simulink model "test_8m_0508"  (R2024a)
settings: Solver=FixedStepAuto  StartTime=0.0  StopTime=30  FixedStep=dt  RelTol=1e-3
values from neighbouring files (symbols this model uses):
  attitude_0 = [0; -90;  -0]    [ini_param_8m_0522.m]
  b = 4.0    (= 4)    [ini_param_8m_0522.m]
  cbar = 0.75    [ini_param_8m_0522.m]
  dt = 0.004    [ini_param_8m_0522.m]
  H = 1000    [ini_param_8m_0522.m]
  N_data = [0,200, 491, 804, 1077, 1344, 1559, 1832, 2078, 2318, 2579,            2864, 3117, 3371, 3608.2, 3872, 4055.7, 4291, 4507, 4739, 4935]'    [cal_motor.m]
  N_pwm = 0.01*[0, 5 ,10 ,15 ,20 ,25 ,30 ,35,40, 45 ,50 ,              55 ,60 ,65 ,70, 75, 80 , 85 ,90 ,95 ,100]'    [cal_motor.m]
  pitch_rate_K = 1    [ini_param_8m_0522.m]
  roll_rate_K = 1    [ini_param_8m_0522.m]
  S = 6.0    (= 6)    [ini_param_8m_0522.m]
  Ts = 0.05    [ini_param_8m_0522.m]
  Ts_sur = 0.25    [ini_param_8m_0522.m]
  yaw_rate_K = 1    [ini_param_8m_0522.m]
undefined symbols (not defined in the file or in its folder): sigbuilder_block, UAV
libraries: slpidlib x9, simulink_extras x6, sharedtransform x2, shared6dof x1
(part 4 of 11)

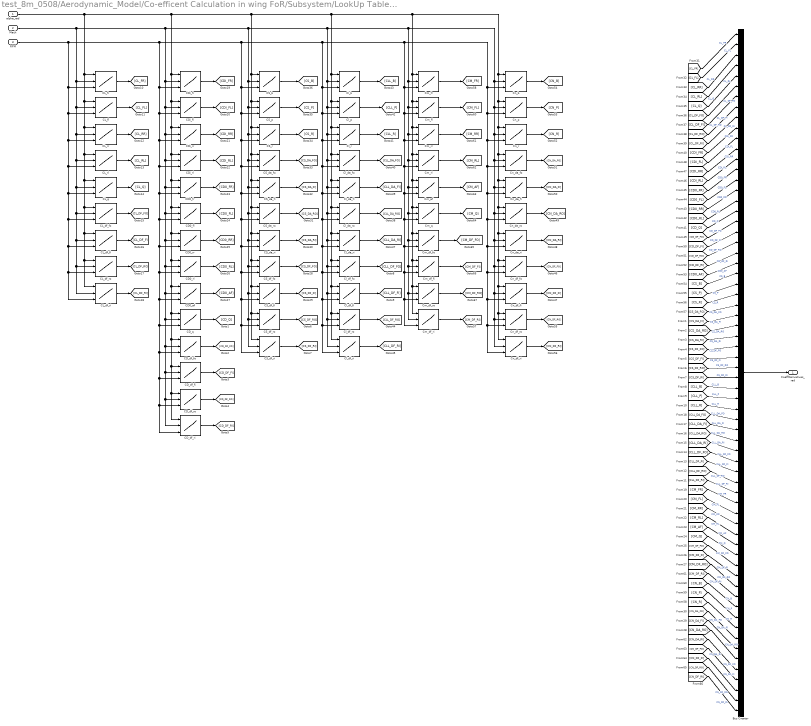
== system test_8m_0508/Aerodynamic_Model/Co-efficent Calculation in wing FoR/Subsystem/LookUp Table for Coeffients_WS1 ==
  alpha_rad : Inport
  Mach : Inport  Port=2
  RPM : Inport  Port=3
  Bus Creator : BusCreator  Inputs=66
  CD0_af : Lookup_n-D  NumberOfTableDimensions=3  DataSpecification=Lookup table object  LookupTableObject=CD0_af  BreakpointsForDimension3=[5, 7]  Table=reshape(repmat([4 5 6;16 19 20;10 18 23],1,2),[3,3,2])  InternalRulePriority=Speed  RndMeth=Simplest
      settings: InputPortMap=u0,u1,u2
  CD0_fl : Lookup_n-D  NumberOfTableDimensions=3  DataSpecification=Lookup table object  LookupTableObject=CD0_fl  BreakpointsForDimension3=[5, 7]  Table=reshape(repmat([4 5 6;16 19 20;10 18 23],1,2),[3,3,2])  InternalRulePriority=Speed  RndMeth=Simplest
      settings: InputPortMap=u0,u1,u2
  CD0_fr : Lookup_n-D  NumberOfTableDimensions=3  DataSpecification=Lookup table object  LookupTableObject=CD0_fr  BreakpointsForDimension3=[5, 7]  Table=reshape(repmat([4 5 6;16 19 20;10 18 23],1,2),[3,3,2])  InternalRulePriority=Speed  RndMeth=Simplest
      settings: InputPortMap=u0,u1,u2
  CD0_rl : Lookup_n-D  NumberOfTableDimensions=3  DataSpecification=Lookup table object  LookupTableObject=CD0_rl  BreakpointsForDimension3=[5, 7]  Table=reshape(repmat([4 5 6;16 19 20;10 18 23],1,2),[3,3,2])  InternalRulePriority=Speed  RndMeth=Simplest
      settings: InputPortMap=u0,u1,u2
  CD0_rr : Lookup_n-D  NumberOfTableDimensions=3  DataSpecification=Lookup table object  LookupTableObject=CD0_rr  BreakpointsForDimension3=[5, 7]  Table=reshape(repmat([4 5 6;16 19 20;10 18 23],1,2),[3,3,2])  InternalRulePriority=Speed  RndMeth=Simplest
      settings: InputPortMap=u0,u1,u2
  CD_df_fi : Lookup_n-D  NumberOfTableDimensions=3  DataSpecification=Lookup table object  LookupTableObject=CD_df_fi  BreakpointsForDimension3=[5, 7]  Table=reshape(repmat([4 5 6;16 19 20;10 18 23],1,2),[3,3,2])  InternalRulePriority=Speed  RndMeth=Simplest
      settings: InputPortMap=u0,u1,u2
  CD_df_fo : Lookup_n-D  NumberOfTableDimensions=3  DataSpecification=Lookup table object  LookupTableObject=CD_df_fo  BreakpointsForDimension3=[5, 7]  Table=reshape(repmat([4 5 6;16 19 20;10 18 23],1,2),[3,3,2])  InternalRulePriority=Speed  RndMeth=Simplest
      settings: InputPortMap=u0,u1,u2
  CD_df_ri : Lookup_n-D  NumberOfTableDimensions=3  DataSpecification=Lookup table object  LookupTableObject=CD_df_ri  BreakpointsForDimension3=[5, 7]  Table=reshape(repmat([4 5 6;16 19 20;10 18 23],1,2),[3,3,2])  InternalRulePriority=Speed  RndMeth=Simplest
      settings: InputPortMap=u0,u1,u2
  CD_df_ro : Lookup_n-D  NumberOfTableDimensions=3  DataSpecification=Lookup table object  LookupTableObject=CD_df_ro  BreakpointsForDimension3=[5, 7]  Table=reshape(repmat([4 5 6;16 19 20;10 18 23],1,2),[3,3,2])  InternalRulePriority=Speed  RndMeth=Simplest
      settings: InputPortMap=u0,u1,u2
  CD_q : Lookup_n-D  NumberOfTableDimensions=3  DataSpecification=Lookup table object  LookupTableObject=CD_q  BreakpointsForDimension3=[5, 7]  Table=reshape(repmat([4 5 6;16 19 20;10 18 23],1,2),[3,3,2])  InternalRulePriority=Speed  RndMeth=Simplest
      settings: InputPortMap=u0,u1,u2
  CDi_fl : Lookup_n-D  NumberOfTableDimensions=3  DataSpecification=Lookup table object  LookupTableObject=CDi_fl  BreakpointsForDimension3=[5, 7]  Table=reshape(repmat([4 5 6;16 19 20;10 18 23],1,2),[3,3,2])  InternalRulePriority=Speed  RndMeth=Simplest
      settings: InputPortMap=u0,u1,u2
  CDi_fr : Lookup_n-D  NumberOfTableDimensions=3  DataSpecification=Lookup table object  LookupTableObject=CDi_fr  BreakpointsForDimension3=[5, 7]  Table=reshape(repmat([4 5 6;16 19 20;10 18 23],1,2),[3,3,2])  InternalRulePriority=Speed  RndMeth=Simplest
      settings: InputPortMap=u0,u1,u2
  CDi_rl : Lookup_n-D  NumberOfTableDimensions=3  DataSpecification=Lookup table object  LookupTableObject=CDi_rl  BreakpointsForDimension3=[5, 7]  Table=reshape(repmat([4 5 6;16 19 20;10 18 23],1,2),[3,3,2])  InternalRulePriority=Speed  RndMeth=Simplest
      settings: InputPortMap=u0,u1,u2
  CDi_rr : Lookup_n-D  NumberOfTableDimensions=3  DataSpecification=Lookup table object  LookupTableObject=CDi_rr  BreakpointsForDimension3=[5, 7]  Table=reshape(repmat([4 5 6;16 19 20;10 18 23],1,2),[3,3,2])  InternalRulePriority=Speed  RndMeth=Simplest
      settings: InputPortMap=u0,u1,u2
  CL_df_fi : Lookup_n-D  NumberOfTableDimensions=3  DataSpecification=Lookup table object  LookupTableObject=CL_df_fi  BreakpointsForDimension3=[5, 7]  Table=reshape(repmat([4 5 6;16 19 20;10 18 23],1,2),[3,3,2])  InternalRulePriority=Speed  RndMeth=Simplest
      settings: InputPortMap=u0,u1,u2
  CL_df_fo : Lookup_n-D  NumberOfTableDimensions=3  DataSpecification=Lookup table object  LookupTableObject=CL_df_fo  BreakpointsForDimension3=[5, 7]  Table=reshape(repmat([4 5 6;16 19 20;10 18 23],1,2),[3,3,2])  InternalRulePriority=Speed  RndMeth=Simplest
      settings: InputPortMap=u0,u1,u2
  CL_df_ri : Lookup_n-D  NumberOfTableDimensions=3  DataSpecification=Lookup table object  LookupTableObject=CL_df_ri  BreakpointsForDimension3=[5, 7]  Table=reshape(repmat([4 5 6;16 19 20;10 18 23],1,2),[3,3,2])  InternalRulePriority=Speed  RndMeth=Simplest
      settings: InputPortMap=u0,u1,u2
  CL_df_ro : Lookup_n-D  NumberOfTableDimensions=3  DataSpecification=Lookup table object  LookupTableObject=CL_df_ro  BreakpointsForDimension3=[5, 7]  Table=reshape(repmat([4 5 6;16 19 20;10 18 23],1,2),[3,3,2])  InternalRulePriority=Speed  RndMeth=Simplest
      settings: InputPortMap=u0,u1,u2
  CL_fl : Lookup_n-D  NumberOfTableDimensions=3  DataSpecification=Lookup table object  LookupTableObject=CL_fl  BreakpointsForDimension3=[5, 7]  Table=reshape(repmat([4 5 6;16 19 20;10 18 23],1,2),[3,3,2])  InternalRulePriority=Speed  RndMeth=Simplest
      settings: InputPortMap=u0,u1,u2
  CL_fr : Lookup_n-D  NumberOfTableDimensions=3  DataSpecification=Lookup table object  LookupTableObject=CL_fr  BreakpointsForDimension3=[5, 7]  Table=reshape(repmat([4 5 6;16 19 20;10 18 23],1,2),[3,3,2])  InternalRulePriority=Speed  RndMeth=Simplest
      settings: InputPortMap=u0,u1,u2
  CL_q : Lookup_n-D  NumberOfTableDimensions=3  DataSpecification=Lookup table object  LookupTableObject=CL_q  BreakpointsForDimension3=[5, 7]  Table=reshape(repmat([4 5 6;16 19 20;10 18 23],1,2),[3,3,2])  InternalRulePriority=Speed  RndMeth=Simplest
      settings: InputPortMap=u0,u1,u2
  CL_rl : Lookup_n-D  NumberOfTableDimensions=3  DataSpecification=Lookup table object  LookupTableObject=CL_rl  BreakpointsForDimension3=[5, 7]  Table=reshape(repmat([4 5 6;16 19 20;10 18 23],1,2),[3,3,2])  InternalRulePriority=Speed  RndMeth=Simplest
      settings: InputPortMap=u0,u1,u2
  CL_rr : Lookup_n-D  NumberOfTableDimensions=3  DataSpecification=Lookup table object  LookupTableObject=CL_rr  BreakpointsForDimension3=[5, 7]  Table=reshape(repmat([4 5 6;16 19 20;10 18 23],1,2),[3,3,2])  InternalRulePriority=Speed  RndMeth=Simplest
      settings: InputPortMap=u0,u1,u2
  CS_b : Lookup_n-D  NumberOfTableDimensions=3  DataSpecification=Lookup table object  LookupTableObject=CS_b  BreakpointsForDimension3=[5, 7]  Table=reshape(repmat([4 5 6;16 19 20;10 18 23],1,2),[3,3,2])  InternalRulePriority=Speed  RndMeth=Simplest
      settings: InputPortMap=u0,u1,u2
  CS_da_fi : Lookup_n-D  NumberOfTableDimensions=3  DataSpecification=Lookup table object  LookupTableObject=CS_da_fi  BreakpointsForDimension3=[5, 7]  Table=reshape(repmat([4 5 6;16 19 20;10 18 23],1,2),[3,3,2])  InternalRulePriority=Speed  RndMeth=Simplest
      settings: InputPortMap=u0,u1,u2
  CS_da_fo : Lookup_n-D  NumberOfTableDimensions=3  DataSpecification=Lookup table object  LookupTableObject=CS_da_fo  BreakpointsForDimension3=[5, 7]  Table=reshape(repmat([4 5 6;16 19 20;10 18 23],1,2),[3,3,2])  InternalRulePriority=Speed  RndMeth=Simplest
      settings: InputPortMap=u0,u1,u2
  CS_da_ri : Lookup_n-D  NumberOfTableDimensions=3  DataSpecification=Lookup table object  LookupTableObject=CS_da_ri  BreakpointsForDimension3=[5, 7]  Table=reshape(repmat([4 5 6;16 19 20;10 18 23],1,2),[3,3,2])  InternalRulePriority=Speed  RndMeth=Simplest
      settings: InputPortMap=u0,u1,u2
  CS_da_ro : Lookup_n-D  NumberOfTableDimensions=3  DataSpecification=Lookup table object  LookupTableObject=CS_da_ro  BreakpointsForDimension3=[5, 7]  Table=reshape(repmat([4 5 6;16 19 20;10 18 23],1,2),[3,3,2])  InternalRulePriority=Speed  RndMeth=Simplest
      settings: InputPortMap=u0,u1,u2
  CS_df_fi : Lookup_n-D  NumberOfTableDimensions=3  DataSpecification=Lookup table object  LookupTableObject=CS_df_fi  BreakpointsForDimension3=[5, 7]  Table=reshape(repmat([4 5 6;16 19 20;10 18 23],1,2),[3,3,2])  InternalRulePriority=Speed  RndMeth=Simplest
      settings: InputPortMap=u0,u1,u2
  CS_df_fo : Lookup_n-D  NumberOfTableDimensions=3  DataSpecification=Lookup table object  LookupTableObject=CS_df_fo  BreakpointsForDimension3=[5, 7]  Table=reshape(repmat([4 5 6;16 19 20;10 18 23],1,2),[3,3,2])  InternalRulePriority=Speed  RndMeth=Simplest
      settings: InputPortMap=u0,u1,u2
  CS_df_ri : Lookup_n-D  NumberOfTableDimensions=3  DataSpecification=Lookup table object  LookupTableObject=CS_df_ri  BreakpointsForDimension3=[5, 7]  Table=reshape(repmat([4 5 6;16 19 20;10 18 23],1,2),[3,3,2])  InternalRulePriority=Speed  RndMeth=Simplest
      settings: InputPortMap=u0,u1,u2
  CS_df_ro : Lookup_n-D  NumberOfTableDimensions=3  DataSpecification=Lookup table object  LookupTableObject=CS_df_ro  BreakpointsForDimension3=[5, 7]  Table=reshape(repmat([4 5 6;16 19 20;10 18 23],1,2),[3,3,2])  InternalRulePriority=Speed  RndMeth=Simplest
      settings: InputPortMap=u0,u1,u2
  CS_p : Lookup_n-D  NumberOfTableDimensions=3  DataSpecification=Lookup table object  LookupTableObject=CS_p  BreakpointsForDimension3=[5, 7]  Table=reshape(repmat([4 5 6;16 19 20;10 18 23],1,2),[3,3,2])  InternalRulePriority=Speed  RndMeth=Simplest
      settings: InputPortMap=u0,u1,u2
  CS_r : Lookup_n-D  NumberOfTableDimensions=3  DataSpecification=Lookup table object  LookupTableObject=CS_r  BreakpointsForDimension3=[5, 7]  Table=reshape(repmat([4 5 6;16 19 20;10 18 23],1,2),[3,3,2])  InternalRulePriority=Speed  RndMeth=Simplest
      settings: InputPortMap=u0,u1,u2
  Cl_b : Lookup_n-D  NumberOfTableDimensions=3  DataSpecification=Lookup table object  LookupTableObject=Cl_b  BreakpointsForDimension3=[5, 7]  Table=reshape(repmat([4 5 6;16 19 20;10 18 23],1,2),[3,3,2])  InternalRulePriority=Speed  RndMeth=Simplest
      settings: InputPortMap=u0,u1,u2
  Cl_da_fi : Lookup_n-D  NumberOfTableDimensions=3  DataSpecification=Lookup table object  LookupTableObject=Cl_da_fi  BreakpointsForDimension3=[5, 7]  Table=reshape(repmat([4 5 6;16 19 20;10 18 23],1,2),[3,3,2])  InternalRulePriority=Speed  RndMeth=Simplest
      settings: InputPortMap=u0,u1,u2
  Cl_da_fo : Lookup_n-D  NumberOfTableDimensions=3  DataSpecification=Lookup table object  LookupTableObject=Cl_da_fo  BreakpointsForDimension3=[5, 7]  Table=reshape(repmat([4 5 6;16 19 20;10 18 23],1,2),[3,3,2])  InternalRulePriority=Speed  RndMeth=Simplest
      settings: InputPortMap=u0,u1,u2
  Cl_da_ri : Lookup_n-D  NumberOfTableDimensions=3  DataSpecification=Lookup table object  LookupTableObject=Cl_da_ri  BreakpointsForDimension3=[5, 7]  Table=reshape(repmat([4 5 6;16 19 20;10 18 23],1,2),[3,3,2])  InternalRulePriority=Speed  RndMeth=Simplest
      settings: InputPortMap=u0,u1,u2
  Cl_da_ro : Lookup_n-D  NumberOfTableDimensions=3  DataSpecification=Lookup table object  LookupTableObject=Cl_da_ro  BreakpointsForDimension3=[5, 7]  Table=reshape(repmat([4 5 6;16 19 20;10 18 23],1,2),[3,3,2])  InternalRulePriority=Speed  RndMeth=Simplest
      settings: InputPortMap=u0,u1,u2
  Cl_df_fi : Lookup_n-D  NumberOfTableDimensions=3  DataSpecification=Lookup table object  LookupTableObject=Cl_df_fi  BreakpointsForDimension3=[5, 7]  Table=reshape(repmat([4 5 6;16 19 20;10 18 23],1,2),[3,3,2])  InternalRulePriority=Speed  RndMeth=Simplest
      settings: InputPortMap=u0,u1,u2
  Cl_df_fo : Lookup_n-D  NumberOfTableDimensions=3  DataSpecification=Lookup table object  LookupTableObject=Cl_df_fo  BreakpointsForDimension3=[5, 7]  Table=reshape(repmat([4 5 6;16 19 20;10 18 23],1,2),[3,3,2])  InternalRulePriority=Speed  RndMeth=Simplest
      settings: InputPortMap=u0,u1,u2
  Cl_df_ri : Lookup_n-D  NumberOfTableDimensions=3  DataSpecification=Lookup table object  LookupTableObject=Cl_df_ri  BreakpointsForDimension3=[5, 7]  Table=reshape(repmat([4 5 6;16 19 20;10 18 23],1,2),[3,3,2])  InternalRulePriority=Speed  RndMeth=Simplest
      settings: InputPortMap=u0,u1,u2
  Cl_df_ro : Lookup_n-D  NumberOfTableDimensions=3  DataSpecification=Lookup table object  LookupTableObject=Cl_df_ro  BreakpointsForDimension3=[5, 7]  Table=reshape(repmat([4 5 6;16 19 20;10 18 23],1,2),[3,3,2])  InternalRulePriority=Speed  RndMeth=Simplest
      settings: InputPortMap=u0,u1,u2
  Cl_p : Lookup_n-D  NumberOfTableDimensions=3  DataSpecification=Lookup table object  LookupTableObject=Cl_p  BreakpointsForDimension3=[5, 7]  Table=reshape(repmat([4 5 6;16 19 20;10 18 23],1,2),[3,3,2])  InternalRulePriority=Speed  RndMeth=Simplest
      settings: InputPortMap=u0,u1,u2
  Cl_r : Lookup_n-D  NumberOfTableDimensions=3  DataSpecification=Lookup table object  LookupTableObject=Cl_r  BreakpointsForDimension3=[5, 7]  Table=reshape(repmat([4 5 6;16 19 20;10 18 23],1,2),[3,3,2])  InternalRulePriority=Speed  RndMeth=Simplest
      settings: InputPortMap=u0,u1,u2
  Cm_af : Lookup_n-D  NumberOfTableDimensions=3  DataSpecification=Lookup table object  LookupTableObject=Cm_af  BreakpointsForDimension3=[5, 7]  Table=reshape(repmat([4 5 6;16 19 20;10 18 23],1,2),[3,3,2])  InternalRulePriority=Speed  RndMeth=Simplest
      settings: InputPortMap=u0,u1,u2
  Cm_df_fi : Lookup_n-D  NumberOfTableDimensions=3  DataSpecification=Lookup table object  LookupTableObject=Cm_df_fi  BreakpointsForDimension3=[5, 7]  Table=reshape(repmat([4 5 6;16 19 20;10 18 23],1,2),[3,3,2])  InternalRulePriority=Speed  RndMeth=Simplest
      settings: InputPortMap=u0,u1,u2
  Cm_df_fo : Lookup_n-D  NumberOfTableDimensions=3  DataSpecification=Lookup table object  LookupTableObject=Cm_df_fo  BreakpointsForDimension3=[5, 7]  Table=reshape(repmat([4 5 6;16 19 20;10 18 23],1,2),[3,3,2])  InternalRulePriority=Speed  RndMeth=Simplest
      settings: InputPortMap=u0,u1,u2
  Cm_df_ri : Lookup_n-D  NumberOfTableDimensions=3  DataSpecification=Lookup table object  LookupTableObject=Cm_df_ri  BreakpointsForDimension3=[5, 7]  Table=reshape(repmat([4 5 6;16 19 20;10 18 23],1,2),[3,3,2])  InternalRulePriority=Speed  RndMeth=Simplest
      settings: InputPortMap=u0,u1,u2
  Cm_df_ro : Lookup_n-D  NumberOfTableDimensions=3  DataSpecification=Lookup table object  LookupTableObject=Cm_df_ro  BreakpointsForDimension3=[5, 7]  Table=reshape(repmat([4 5 6;16 19 20;10 18 23],1,2),[3,3,2])  InternalRulePriority=Speed  RndMeth=Simplest
      settings: InputPortMap=u0,u1,u2
  Cm_fl : Lookup_n-D  NumberOfTableDimensions=3  DataSpecification=Lookup table object  LookupTableObject=Cm_fl  BreakpointsForDimension3=[5, 7]  Table=reshape(repmat([4 5 6;16 19 20;10 18 23],1,2),[3,3,2])  InternalRulePriority=Speed  RndMeth=Simplest
      settings: InputPortMap=u0,u1,u2
  Cm_fr : Lookup_n-D  NumberOfTableDimensions=3  DataSpecification=Lookup table object  LookupTableObject=Cm_fr  BreakpointsForDimension3=[5, 7]  Table=reshape(repmat([4 5 6;16 19 20;10 18 23],1,2),[3,3,2])  InternalRulePriority=Speed  RndMeth=Simplest
      settings: InputPortMap=u0,u1,u2
  Cm_q : Lookup_n-D  NumberOfTableDimensions=3  DataSpecification=Lookup table object  LookupTableObject=Cm_q  BreakpointsForDimension3=[5, 7]  Table=reshape(repmat([4 5 6;16 19 20;10 18 23],1,2),[3,3,2])  InternalRulePriority=Speed  RndMeth=Simplest
      settings: InputPortMap=u0,u1,u2
  Cm_rl : Lookup_n-D  NumberOfTableDimensions=3  DataSpecification=Lookup table object  LookupTableObject=Cm_rl  BreakpointsForDimension3=[5, 7]  Table=reshape(repmat([4 5 6;16 19 20;10 18 23],1,2),[3,3,2])  InternalRulePriority=Speed  RndMeth=Simplest
      settings: InputPortMap=u0,u1,u2
  Cm_rr : Lookup_n-D  NumberOfTableDimensions=3  DataSpecification=Lookup table object  LookupTableObject=Cm_rr  BreakpointsForDimension3=[5, 7]  Table=reshape(repmat([4 5 6;16 19 20;10 18 23],1,2),[3,3,2])  InternalRulePriority=Speed  RndMeth=Simplest
      settings: InputPortMap=u0,u1,u2
  Cn_b : Lookup_n-D  NumberOfTableDimensions=3  DataSpecification=Lookup table object  LookupTableObject=Cn_b  BreakpointsForDimension3=[5, 7]  Table=reshape(repmat([4 5 6;16 19 20;10 18 23],1,2),[3,3,2])  InternalRulePriority=Speed  RndMeth=Simplest
      settings: InputPortMap=u0,u1,u2
  Cn_da_fi : Lookup_n-D  NumberOfTableDimensions=3  DataSpecification=Lookup table object  LookupTableObject=Cn_da_fi  BreakpointsForDimension3=[5, 7]  Table=reshape(repmat([4 5 6;16 19 20;10 18 23],1,2),[3,3,2])  InternalRulePriority=Speed  RndMeth=Simplest
      settings: InputPortMap=u0,u1,u2
  Cn_da_fo : Lookup_n-D  NumberOfTableDimensions=3  DataSpecification=Lookup table object  LookupTableObject=Cn_da_fo  BreakpointsForDimension3=[5, 7]  Table=reshape(repmat([4 5 6;16 19 20;10 18 23],1,2),[3,3,2])  InternalRulePriority=Speed  RndMeth=Simplest
      settings: InputPortMap=u0,u1,u2
  Cn_da_ri : Lookup_n-D  NumberOfTableDimensions=3  DataSpecification=Lookup table object  LookupTableObject=Cn_da_ri  BreakpointsForDimension3=[5, 7]  Table=reshape(repmat([4 5 6;16 19 20;10 18 23],1,2),[3,3,2])  InternalRulePriority=Speed  RndMeth=Simplest
      settings: InputPortMap=u0,u1,u2
  Cn_da_ro : Lookup_n-D  NumberOfTableDimensions=3  DataSpecification=Lookup table object  LookupTableObject=Cn_da_ro  BreakpointsForDimension3=[5, 7]  Table=reshape(repmat([4 5 6;16 19 20;10 18 23],1,2),[3,3,2])  InternalRulePriority=Speed  RndMeth=Simplest
      settings: InputPortMap=u0,u1,u2
  Cn_df_fi : Lookup_n-D  NumberOfTableDimensions=3  DataSpecification=Lookup table object  LookupTableObject=Cn_df_fi  BreakpointsForDimension3=[5, 7]  Table=reshape(repmat([4 5 6;16 19 20;10 18 23],1,2),[3,3,2])  InternalRulePriority=Speed  RndMeth=Simplest
      settings: InputPortMap=u0,u1,u2
  Cn_df_fo : Lookup_n-D  NumberOfTableDimensions=3  DataSpecification=Lookup table object  LookupTableObject=Cn_df_fo  BreakpointsForDimension3=[5, 7]  Table=reshape(repmat([4 5 6;16 19 20;10 18 23],1,2),[3,3,2])  InternalRulePriority=Speed  RndMeth=Simplest
      settings: InputPortMap=u0,u1,u2
  Cn_df_ri : Lookup_n-D  NumberOfTableDimensions=3  DataSpecification=Lookup table object  LookupTableObject=Cn_df_ri  BreakpointsForDimension3=[5, 7]  Table=reshape(repmat([4 5 6;16 19 20;10 18 23],1,2),[3,3,2])  InternalRulePriority=Speed  RndMeth=Simplest
      settings: InputPortMap=u0,u1,u2
  Cn_df_ro : Lookup_n-D  NumberOfTableDimensions=3  DataSpecification=Lookup table object  LookupTableObject=Cn_df_ro  BreakpointsForDimension3=[5, 7]  Table=reshape(repmat([4 5 6;16 19 20;10 18 23],1,2),[3,3,2])  InternalRulePriority=Speed  RndMeth=Simplest
      settings: InputPortMap=u0,u1,u2
  Cn_p : Lookup_n-D  NumberOfTableDimensions=3  DataSpecification=Lookup table object  LookupTableObject=Cn_p  BreakpointsForDimension3=[5, 7]  Table=reshape(repmat([4 5 6;16 19 20;10 18 23],1,2),[3,3,2])  InternalRulePriority=Speed  RndMeth=Simplest
      settings: InputPortMap=u0,u1,u2
  Cn_r : Lookup_n-D  NumberOfTableDimensions=3  DataSpecification=Lookup table object  LookupTableObject=Cn_r  BreakpointsForDimension3=[5, 7]  Table=reshape(repmat([4 5 6;16 19 20;10 18 23],1,2),[3,3,2])  InternalRulePriority=Speed  RndMeth=Simplest
      settings: InputPortMap=u0,u1,u2
  CoeffDerivatives_rad : Outport
  wires:
  Bus Creator/1 -> CoeffDerivatives_rad/1
  [CD_DF_FO] -> Bus Creator/19  "CD_DF_FO"
  [CL_Q] -> Bus Creator/5  "CL_Q"
  [CL_RL] -> Bus Creator/4  "CL_RL"
  [CS_B] -> Bus Creator/24  "CS_B"
  [CD0_AF] -> Bus Creator/23  "CD0_AF"
  [CD_DF_FI] -> Bus Creator/20  "CD_DF_FI"
  [CD_Q] -> Bus Creator/18  "CD_Q"
  [CDI_FL] -> Bus Creator/11  "CDI_FL"
  [CL_DF_RI] -> Bus Creator/9  "CL_DF_RI"
  [CD0_FL] -> Bus Creator/15  "CD0_FL"
  [CD0_RL] -> Bus Creator/17  "CD0_RL"
  [CL_FR] -> Bus Creator/1  "CL_FR"
  [CD0_FR] -> Bus Creator/14  "CD0_FR"
  [CDI_FR] -> Bus Creator/10  "CDI_FR"
  [CDI_RL] -> Bus Creator/13  "CDI_RL"
  [CS_R] -> Bus Creator/26  "CS_R"
  [CDI_RR] -> Bus Creator/12  "CDI_RR"
  [CL_RR] -> Bus Creator/3  "CL_RR"
  [CL_DF_FI] -> Bus Creator/7  "CL_DF_FI"
  [CD_DF_RO] -> Bus Creator/21  "CD_DF_RO"
  [CD_DF_RI] -> Bus Creator/22  "CD_DF_RI"
  [CL_DF_FO] -> Bus Creator/6  "CL_DF_FO"
  [CS_DA_FO] -> Bus Creator/27  "CS_DA_FO"
  [CD0_RR] -> Bus Creator/16  "CD0_RR"
  [CS_P] -> Bus Creator/25  "CS_P"
  [CL_DF_RO] -> Bus Creator/8  "CL_DF_RO"
  [CL_FL] -> Bus Creator/2  "CL_FL"
  CL_fr/1 -> [CL_FR]
  CL_fl/1 -> [CL_FL]
  CL_rr/1 -> [CL_RR]
  CL_rl/1 -> [CL_RL]
  CL_q/1 -> [CL_Q]
  CL_df_fo/1 -> [CL_DF_FO]
  CL_df_fi/1 -> [CL_DF_FI]
  CL_df_ro/1 -> [CL_DF_RO]
  CL_df_ri/1 -> [CL_DF_RI]
  CDi_fr/1 -> [CDI_FR]
  CDi_fl/1 -> [CDI_FL]
  CDi_rr/1 -> [CDI_RR]
  CDi_rl/1 -> [CDI_RL]
  CD0_fr/1 -> [CD0_FR]
  CD0_fl/1 -> [CD0_FL]
  CD0_rr/1 -> [CD0_RR]
  CD0_rl/1 -> [CD0_RL]
  CD0_af/1 -> [CD0_AF]
  CD_q/1 -> [CD_Q]
  CD_df_fo/1 -> [CD_DF_FO]
  CD_df_fi/1 -> [CD_DF_FI]
  CS_b/1 -> [CS_B]
  CS_p/1 -> [CS_P]
  CS_r/1 -> [CS_R]
  CS_da_fo/1 -> [CS_DA_FO]
  CS_da_fi/1 -> [CS_DA_FI]
  CS_da_ro/1 -> [CS_DA_RO]
  CS_da_ri/1 -> [CS_DA_RI]
  CS_df_fo/1 -> [CS_DF_FO]
  CS_df_fi/1 -> [CS_DF_FI]
  CS_df_ro/1 -> [CS_DF_RO]
  CS_df_ri/1 -> [CS_DF_RI]
  Cl_b/1 -> [CLL_B]
  Cl_p/1 -> [CLL_P]
  Cl_r/1 -> [CLL_R]
  Cl_da_fo/1 -> [CLL_DA_FO]
  Cl_da_fi/1 -> [CLL_DA_FI]
  Cl_da_ro/1 -> [CLL_DA_RO]
  Cl_da_ri/1 -> [CLL_DA_RI]
  Cl_df_fo/1 -> [CLL_DF_FO]
  Cl_df_fi/1 -> [CLL_DF_FI]
  Cl_df_ro/1 -> [CLL_DF_RO]
  Cl_df_ri/1 -> [CLL_DF_RI]
  Cm_fr/1 -> [CM_FR]
  Cm_fl/1 -> [CM_FL]
  Cm_rr/1 -> [CM_RR]
  Cm_rl/1 -> [CM_RL]
  Cm_af/1 -> [CM_AF]
  Cm_q/1 -> [CM_Q]
  Cm_df_fo/1 -> [CM_DF_FO]
  Cm_df_fi/1 -> [CM_DF_FI]
  Cm_df_ro/1 -> [CM_DF_RO]
  Cm_df_ri/1 -> [CM_DF_RI]
  Cn_b/1 -> [CN_B]
  Cn_p/1 -> [CN_P]
  Cn_r/1 -> [CN_R]
  Cn_da_fo/1 -> [CN_DA_FO]
  Cn_da_fi/1 -> [CN_DA_FI]
  Cn_da_ro/1 -> [CN_DA_RO]
  Cn_da_ri/1 -> [CN_DA_RI]
  Cn_df_fo/1 -> [CN_DF_FO]
  Cn_df_fi/1 -> [CN_DF_FI]
  Cn_df_ro/1 -> [CN_DF_RO]
  Cn_df_ri/1 -> [CN_DF_RI]
  CD_df_ro/1 -> [CD_DF_RO]
  CD_df_ri/1 -> [CD_DF_RI]
  alpha_rad/1 -> CL_df_ri/1, CL_df_ro/1, CL_df_fi/1, CL_df_fo/1, CL_q/1, CL_rl/1, CL_rr/1, CL_fl/1, CL_fr/1, CS_df_ri/1, CS_df_ro/1, CS_df_fi/1, CS_df_fo/1, CS_da_ri/1, CS_da_ro/1, CS_da_fi/1, CS_da_fo/1, CS_r/1, CS_p/1, CS_b/1, Cl_df_ri/1, Cl_df_ro/1, Cl_df_fi/1, Cl_df_fo/1, Cl_da_ri/1, Cl_da_ro/1, Cl_da_fi/1, Cl_da_fo/1, Cl_r/1, Cl_p/1, Cl_b/1, Cn_df_ri/1, Cn_df_ro/1, Cn_df_fi/1, Cn_df_fo/1, Cn_da_ri/1, Cn_da_ro/1, Cn_da_fi/1, Cn_da_fo/1, Cn_r/1, Cn_p/1, Cn_b/1, Cm_df_ri/1, Cm_df_ro/1, Cm_df_fi/1, Cm_df_fo/1, Cm_q/1, Cm_af/1, Cm_rl/1, Cm_rr/1, Cm_fl/1, Cm_fr/1, CD_df_ri/1, CD_df_ro/1, CD_df_fi/1, CD_df_fo/1, CD_q/1, CD0_af/1, CD0_rl/1, CD0_rr/1, CD0_fl/1, CD0_fr/1, CDi_rl/1, CDi_rr/1, CDi_fl/1, CDi_fr/1
  Mach/1 -> CL_df_ri/2, CL_df_ro/2, CL_df_fi/2, CL_df_fo/2, CL_q/2, CL_rl/2, CL_rr/2, CL_fl/2, CL_fr/2, Cn_df_ri/2, Cn_df_ro/2, Cn_df_fi/2, Cn_df_fo/2, Cn_da_ri/2, Cn_da_ro/2, Cn_da_fi/2, Cn_da_fo/2, Cn_r/2, Cn_p/2, Cn_b/2, Cm_df_ri/2, Cm_df_ro/2, Cm_df_fi/2, Cm_df_fo/2, Cm_q/2, Cm_af/2, Cm_rl/2, Cm_rr/2, Cm_fl/2, Cm_fr/2, Cl_df_ri/2, Cl_df_ro/2, Cl_df_fi/2, Cl_df_fo/2, Cl_da_ri/2, Cl_da_ro/2, Cl_da_fi/2, Cl_da_fo/2, Cl_r/2, Cl_p/2, Cl_b/2, CS_df_ri/2, CS_df_ro/2, CS_df_fi/2, CS_df_fo/2, CS_da_ri/2, CS_da_ro/2, CS_da_fi/2, CS_da_fo/2, CS_r/2, CS_p/2, CS_b/2, CD_df_ri/2, CD_df_ro/2, CD_df_fi/2, CD_df_fo/2, CD_q/2, CD0_af/2, CD0_rl/2, CD0_rr/2, CD0_fl/2, CD0_fr/2, CDi_rl/2, CDi_rr/2, CDi_fl/2, CDi_fr/2
  RPM/1 -> Cn_da_ro/3, Cn_df_ri/3, Cn_df_ro/3, Cn_df_fi/3, Cn_df_fo/3, Cn_da_ri/3, Cn_da_fi/3, Cn_da_fo/3, Cn_r/3, Cn_p/3, Cn_b/3, Cm_df_ri/3, Cm_df_ro/3, Cm_df_fi/3, Cm_df_fo/3, Cm_q/3, Cm_af/3, Cm_rl/3, Cm_rr/3, Cm_fl/3, Cm_fr/3, Cl_df_ri/3, Cl_df_ro/3, Cl_df_fi/3, Cl_df_fo/3, Cl_da_ri/3, Cl_da_ro/3, Cl_da_fi/3, Cl_da_fo/3, Cl_r/3, Cl_p/3, Cl_b/3, CS_df_ri/3, CS_df_ro/3, CS_df_fi/3, CS_df_fo/3, CS_da_ri/3, CS_da_ro/3, CS_da_fi/3, CS_da_fo/3, CS_r/3, CS_p/3, CS_b/3, CD_df_ri/3, CD_df_ro/3, CD_df_fi/3, CD_df_fo/3, CD_q/3, CD0_af/3, CD0_rl/3, CD0_rr/3, CD0_fl/3, CD0_fr/3, CDi_rl/3, CDi_rr/3, CDi_fl/3, CDi_fr/3, CL_df_ri/3, CL_df_ro/3, CL_df_fi/3, CL_df_fo/3, CL_q/3, CL_rl/3, CL_rr/3, CL_fl/3, CL_fr/3
  [CS_DA_FI] -> Bus Creator/28  "CS_DA_FI"
  [CS_DA_RO] -> Bus Creator/29  "CS_DA_RO"
  [CS_DA_RI] -> Bus Creator/30  "CS_DA_RI"
  [CS_DF_FO] -> Bus Creator/31  "CS_DF_FO"
  [CS_DF_FI] -> Bus Creator/32  "CS_DF_FI"
  [CS_DF_RO] -> Bus Creator/33  "CS_DF_RO"
  [CS_DF_RI] -> Bus Creator/34  "CS_DF_RI"
  [CLL_B] -> Bus Creator/35  "CLL_B"
  [CLL_P] -> Bus Creator/36  "CLL_P"
  [CLL_R] -> Bus Creator/37  "CLL_R"
  [CLL_DA_FO] -> Bus Creator/38  "CLL_DA_FO"
  [CLL_DA_FI] -> Bus Creator/39  "CLL_DA_FI"
  [CLL_DA_RO] -> Bus Creator/40  "CLL_DA_RO"
  [CLL_DA_RI] -> Bus Creator/41  "CLL_DA_RI"
  [CLL_DF_FO] -> Bus Creator/42  "CLL_DF_FO"
  [CLL_DF_FI] -> Bus Creator/43  "CLL_DF_FI"
  [CLL_DF_RO] -> Bus Creator/44  "CLL_DF_RO"
  [CLL_DF_RI] -> Bus Creator/45  "CLL_DF_RI"
  [CM_FR] -> Bus Creator/46  "CM_FR"
  [CM_FL] -> Bus Creator/47  "CM_FL"
  [CM_RR] -> Bus Creator/48  "CM_RR"
  [CM_RL] -> Bus Creator/49  "CM_RL"
  [CM_AF] -> Bus Creator/50  "CM_AF"
  [CM_Q] -> Bus Creator/51  "CM_Q"
  [CM_DF_FO] -> Bus Creator/52  "CM_DF_FO"
  [CM_DF_FI] -> Bus Creator/53  "CM_DF_FI"
  [CM_DF_RO] -> Bus Creator/54  "CM_DF_RO"
  [CM_DF_RI] -> Bus Creator/55  "CM_DF_RI"
  [CN_B] -> Bus Creator/56  "CN_B"
  [CN_P] -> Bus Creator/57  "CN_P"
  [CN_R] -> Bus Creator/58  "CN_R"
  [CN_DA_FO] -> Bus Creator/59  "CN_DA_FO"
  [CN_DA_FI] -> Bus Creator/60  "CN_DA_FI"
  [CN_DA_RO] -> Bus Creator/61  "CN_DA_RO"
  [CN_DA_RI] -> Bus Creator/62  "CN_DA_RI"
  [CN_DF_FO] -> Bus Creator/63  "CN_DF_FO"
  [CN_DF_FI] -> Bus Creator/64  "CN_DF_FI"
  [CN_DF_RO] -> Bus Creator/65  "CN_DF_RO"
  [CN_DF_RI] -> Bus Creator/66  "CN_DF_RI"
